simulink model "Esempio1NAMU97_OK"  (R2022a)
settings: Solver=ode3  StartTime=0.0  StopTime=1000  RelTol=1e-3  EnableMultiTasking=on
libraries: neural x1
settings Model: Creator=C.Perri  LastModifiedBy=david.naso
settings SolverCC: AlgebraicLoopSolver=TrustRegion
settings DataIOCC: LimitDataPoints=on  SaveFormat=Array  SignalLoggingSaveFormat=ModelDataLogs  ReturnWorkspaceOutputs=off
settings OptimizationCC: InitFltsAndDblsToZero=on  LifeSpan=inf
settings DebuggingCC: SaveWithParameterizedLinksMsg=none  UnderspecifiedInitializationDetection=Classic  MergeDetectMultiDrivingBlocksExec=none  SignalResolutionControl=TryResolveAllWithWarning  SolverPrmCheckMsg=warning  MultiTaskDSMMsg=warning  MultiTaskCondExecSysMsg=none  FcnCallInpInsideContextMsg=warning  UnconnectedInputMsg=warning  UnconnectedOutputMsg=warning  UnconnectedLineMsg=warning  SFUnexpectedBacktrackingDiag=warning  SFNoUnconditionalDefaultTransitionDiag=warning  SFExecutionAtInitializationDiag=none  SFMachineParentedDataDiag=warning  ArithmeticOperatorsInVariantConditions=warning
settings HardwareCC: ProdBitPerPointer=32  ProdBitPerSizeT=32  ProdBitPerPtrDiffT=32  ProdLargestAtomicFloat=None  ProdIntDivRoundTo=Undefined  ProdEndianess=Unspecified  ProdWordSize=32  ProdHWDeviceType=32-bit Generic
settings ModelReferenceCC: PropagateSignalLabelsOutOfModel=off
settings CodeAppCC: StateflowObjectComments=on
settings GRTTargetCC: TargetFcnLib=ansi_tfl_tmw.mat  TargetLangStandard=C89/C90 (ANSI)  CombineOutputUpdateFcns=off  GRTInterface=on
settings ConfigComp: CovMetricSettings=dw  CovSaveCumulativeToWorkspaceVar=on  CovSaveSingleToWorkspaceVar=on

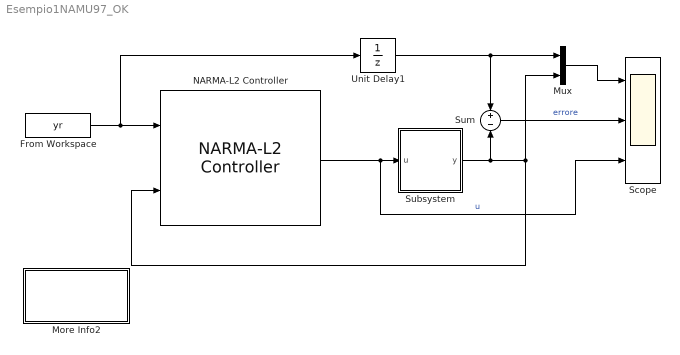
== system Esempio1NAMU97_OK ==
  From Workspace : FromWorkspace  VariableName=yr  SampleTime=1
  More Info2 : Subsystem
      settings: OpenFcn=t=0:1000;y=2*sin(2*pi*t/50)+2*sin(2*pi*t/100);yr=[t' y']; warning off;
      mask Display: disp('Clicca per\ngenerare setpoint yr')
  Mux : Mux  Inputs=2
  NARMA-L2 Controller : neural/Control Systems/NARMA-L2 Controller  Normalize=0  IW1_1=[0.42630333414970916772 0.21731094482351581698 -2.4594992377962321406;-1.1250042834890112697 -1.315085454879722171 -1.9061755760594918385;-2.3953127308528729955 -0.26789106395162498586 -2.1851530204808486957;2.8886495531316684904 0.019930124471541833808 3.3524427736790478605;-2.0453560368104861666 -0.87287435276127345318 3.5384928315645121089;-2.0966657226756790777 -0.46977568072950526279 -1.0196294628291346918;-1.8942840060850905104 0.62011205064125796138 -3.011754286914722023;1.0832101015544206568 -0.060730161198285420587 1.2738833803403237788;1.6620205073373282012 0.43155751039868872621 2.2891478114260266352;-0.69057625355548502011 0.1325858479600546258 -0.77406313103333168613;-0.18252749822169495042 -1.8445385922215771224 -2.8843206942458525788;-0.23618086419646311391 0.28087514242249261853 -1.504741883884554543;-2.7022157676884455135 -1.5985169304653266131 1.5806423520053296539;-0.39850695410066067081 -0.16305224068483864519 1.8719508268500415493;-0.76371416912653478093 0.623107404989408864 1.9149883913076723996]  IW3_2=[1.2439400624745089452 0.12819982625317663527 1.294120585387701805;2.3134360816771244451 0.87839041676604667774 3.4583999519334680528;-0.041016666645749308429 2.2644472610345127706 1.8362931350578701739;-1.1196846665840602952 3.6912367401706762671 0.54161722629641761984;-2.9724621543016249703 -0.76261420006914482084 -2.8996403875718930188;-0.75158937104010625774 2.8976116429132363628 0.45410644083305223839;0.0089331155235166104234 -1.5749851273181265654 2.10197465948123563;-2.7102351996200719775 0.31156611295930131122 -1.5140847686323872789;-1.3728895314999989274 -2.3178154652947662306 3.4096474641809031425;3.7487117077135927445 0.88053531508135851613 -1.4293524916356068477;0.88254719161012706863 1.7603139335295854284 -1.8638721316511182025;-2.7958698742806866733 -0.50154506809153076574 -0.24058160495371880283;-1.0942312757432997028 -1.653220919364879693 -2.9311433776487385572;-3.602235804368768779 0.19687391190821246223 0.5794718565396602683;0.69814250592477222757 0.080691321397038273666 0.082151589294170102029]  IW5_3=-0.81199524878887618939  LW2_1=[0.045918942840653460824 0.51393687452474134947 0.56684732830175255103 -0.52410377499631566334 1.2706990943316247566 0.8754181564353452627 2.5214725573677241321 -0.51325402138344911052 -0.40702984003661052403 -3.2149922160467183652 -1.7982159869064204827 -5.0971377359599436829 -1.4658856802432558286 0.33106531099739838764 1.3815917673706721303]  LW4_3=[1.4124985429593017727 0.22411535948257629847 0.76624774292561015354 1.9719641825254690115 -2.0809613098551036359 -3.6901100810220790471 0.88678216151879019069 -2.3144772450601260871 -1.7023837825694574377 -1.8752716093653194473 -0.054277344743017562345 0.61593509343430397074 1.1509070111030321737 -0.29472750343704801068 -2.5682425656916154644]  LW5_4=-0.85698573790881038548  LW6_5=0.81192570872417135774  LW6_2=-0.31084065039657915452  B1=[-3.3586622665205640992;-2.0046282410854736611;-2.0028632045404100026;-2.1776789764443069686;-1.5057829902394495036;-0.40816324034581275004;-0.10391508495900861342;-0.20487231542973671772;0.054829135605544823684;-2.3312964676425305122;-0.42648611789572127284;0.94117009584237865116;-2.228635089517102319;-3.2413105241987225646;3.9203233920027082959]  B2=-0.15608364254916357039  B3=[4.6677728244043912298;2.4403598421457113332;1.9967152084702803894;0.68334824973412333637;-0.7665478373267708978;-0.7494043185184839917;-1.3048172819592471772;1.6714078297810806006;2.5074864237705694059;1.1045880719597702679;0.14115725787175908978;-2.1623326477721929173;1.5642875799019204663;-2.5682801680551063939;-1.7383728265256981338]  B4=6.9544154148993033715  Limit_output=1  min_output=-7  max_output=7  Use_Previous_Weights=1  Ts=1  S1=15  Ni=2  Nj=2  sim_file=PlantEsempio1  trainfun=trainlm  Use_validation=1  Use_Testing=0  max_i=1  min_i=-1  max_i_int=10  min_i_int=2  sam_training=500  epochs=200  minp=-0.91540440417091439862  maxp=0.9951206990243781636  mint=-5.6694548661466788175  maxt=0.9951206990243781636
      settings: SourceProductBaseCode=NN
  Scope : Scope  NumInputPorts=3
  Subsystem : Subsystem
  Sum : Sum  Inputs=+-
  Unit Delay1 : UnitDelay
  wires:
  Mux/1 -> Scope/1
  From Workspace/1 -> NARMA-L2 Controller/1, Unit Delay1/1
  NARMA-L2 Controller/1 -> Subsystem/1(u), Scope/3  "u"
  Subsystem/1(y) -> Mux/2, NARMA-L2 Controller/2, Sum/2
  Sum/1 -> Scope/2  "errore"
  Unit Delay1/1 -> Sum/1, Mux/1

== system Esempio1NAMU97_OK/More Info2 ==

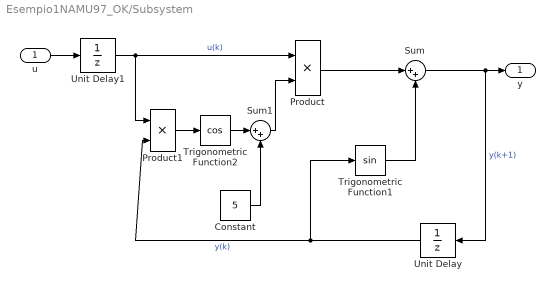
== system Esempio1NAMU97_OK/Subsystem ==
  u : Inport
  Constant : Constant  Value=5
  Product : Product  RndMeth=Zero
  Product1 : Product  RndMeth=Zero
  Sum : Sum  Inputs=|++
  Sum1 : Sum  Inputs=|++
  Trigonometric Function1 : Trigonometry
  Trigonometric Function2 : Trigonometry  Operator=cos
  Unit Delay : UnitDelay
  Unit Delay1 : UnitDelay
  y : Outport
  wires:
  Unit Delay/1 -> Trigonometric Function1/1, Product1/2  "y(k)"
  Product/1 -> Sum/1
  Trigonometric Function1/1 -> Sum/2
  Sum/1 -> Unit Delay/1, y/1  "y(k+1)"
  u/1 -> Unit Delay1/1
  Product1/1 -> Trigonometric Function2/1
  Trigonometric Function2/1 -> Sum1/1
  Sum1/1 -> Product/2
  Constant/1 -> Sum1/2
  Unit Delay1/1 -> Product1/1, Product/1  "u(k)"
